simulink model "InertiaWheelSystemSF"
settings: Solver=ode45  StartTime=0.0  StopTime=10.0  RelTol=1e-6
values from neighbouring files (symbols this model uses):
  A = [0 1 0; a 0 0; 0 0 0]    [modelinertia.m]    (also in modellinertia.m = [0 1 0 0; a 0 0 0; 0 0 0 1; 0 0 0 0]; modellinertia2.m = [0 1 0 0; a 0 0 0; 0 0 0 1; 0 0 0 0])
  ang = [1 0 0]    [modelinertia.m]
  B = [B_tau B_d]    [modelinertia.m]    (also in modellinertia.m = [0; b1; 0; -b2]; modellinertia2.m)
  C = Call    [modelinertia.m]    (also in modellinertia.m = [1 0 0 0]; modellinertia2.m = [1 0 0 0])
  D = zeros(3,2)    [modelinertia.m]    (also in modellinertia.m = 0; modellinertia2.m = 0)
  ki = 1/20    (= 0.05)    [modelinertia.m]
  Kt = 59.1186    [Cindesign.m]
  L = 0.30    (= 0.3)    [modelinertia.m]    (also in modellinertia.m; modellinertia2.m)
  N = 328.9617    [Cindesign.m]
  Tdt = 4.4053    [Cindesign.m]
  Tit = 72.0271    [Cindesign.m]
  x10 = 0    [SysInit.m]
  x20 = 0    [SysInit.m]
  x30 = 0    [SysInit.m]
libraries: simulink x7, cstblocks x2
settings Model: Creator=elt11jke  LastModifiedBy=frt090_B
settings DataIOCC: LimitDataPoints=on  SaveFormat=Array  SignalLoggingSaveFormat=ModelDataLogs  ReturnWorkspaceOutputs=off
settings OptimizationCC: ExpressionDepthLimit=2147483647  LifeSpan=inf  SimCompilerOptimization=Off
settings DebuggingCC: UnderspecifiedInitializationDetection=Classic  MergeDetectMultiDrivingBlocksExec=none  SolverPrmCheckMsg=warning  MultiTaskDSMMsg=warning  MultiTaskCondExecSysMsg=none  FcnCallInpInsideContextMsg=Enable All  FrameProcessingCompatibilityMsg=warning  StateNameClashWarn=warning  StrictBusMsg=None  SFUnexpectedBacktrackingDiag=warning  SFNoUnconditionalDefaultTransitionDiag=warning
settings HardwareCC: ProdBitPerPointer=32  ProdLargestAtomicFloat=None  ProdIntDivRoundTo=Undefined  ProdEndianess=Unspecified  ProdWordSize=32  ProdHWDeviceType=32-bit Generic
settings ModelReferenceCC: PropagateSignalLabelsOutOfModel=off
settings SFSimCC: SimUseLocalCustomCode=off
settings RTWCC: RTWUseLocalCustomCode=off  IncludeERTFirstTime=on  RTWCompilerOptimization=Off
settings GRTTargetCC: GeneratePreprocessorConditionals=Disable all

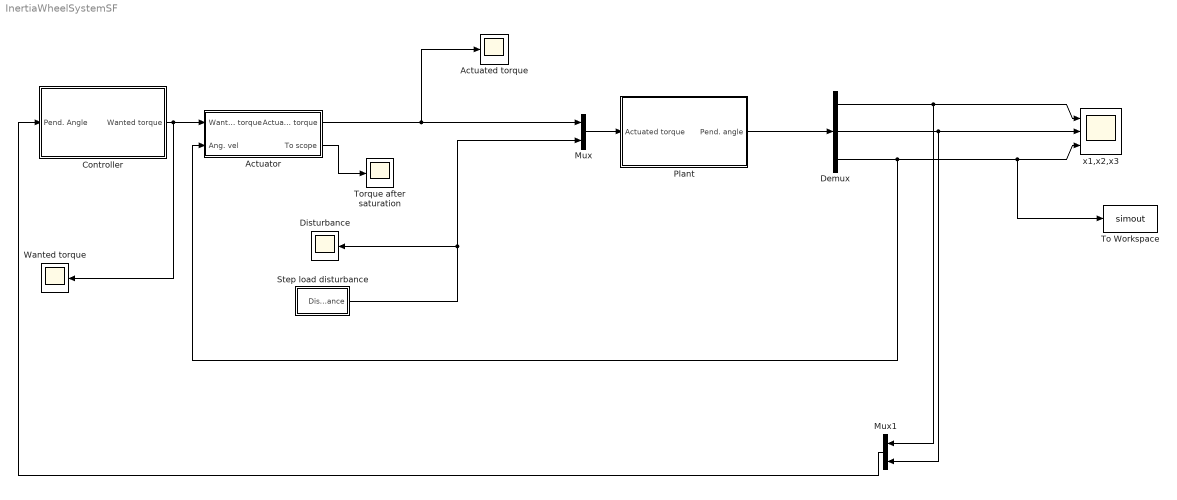
== system InertiaWheelSystemSF ==
  Actuated torque : Scope
      settings: ShowLegends=on  TimeRange=10  YMin=0  YMax=0.00325
  Actuator : Subsystem  TreatAsAtomicUnit=on
  Controller : Subsystem  TreatAsAtomicUnit=on
  Demux : Demux  Outputs=3
  Disturbance : Scope
      settings: ShowLegends=on  TimeRange=10  YMin=-0.01  YMax=0.02  SaveName=ScopeData2
  Mux : Mux  Inputs=2
  Mux1 : Mux  Inputs=2
  Plant : Subsystem  TreatAsAtomicUnit=on
  Step load disturbance : Subsystem
  To Workspace : ToWorkspace  VariableName=simout  SampleTime=-1  SaveFormat=Timeseries
  Torque after saturation : Scope
      settings: ShowLegends=on  TimeRange=10  YMin=0.3648  YMax=0.4032  SaveName=ScopeData4
  Wanted torque : Scope
      settings: ShowLegends=on  TimeRange=10  YMin=-1.355e+07  YMax=-1.3275e+07  SaveName=ScopeData3
  x1,x2,x3 : Scope  NumInputPorts=3
      settings: ShowLegends=on  TimeRange=10  YMin=-6e+38~-6e+39~-20  YMax=2e+38~0~20
  wires:
  Demux/1 -> x1,x2,x3/1, Mux1/1
  Demux/2 -> x1,x2,x3/2, Mux1/2
  Demux/3 -> To Workspace/1, x1,x2,x3/3, Actuator/2(Ang. vel)
  Actuator/2(To scope) -> Torque after saturation/1
  Actuator/1(Actuated torque) -> Mux/1, Actuated torque/1
  Step load disturbance/1(Disturbance) -> Mux/2, Disturbance/1
  Controller/1(Wanted torque) -> Actuator/1(Wanted torque), Wanted torque/1
  Mux/1 -> Plant/1(Actuated torque)
  Plant/1(Pend. angle) -> Demux/1
  Mux1/1 -> Controller/1(Pend. Angle)

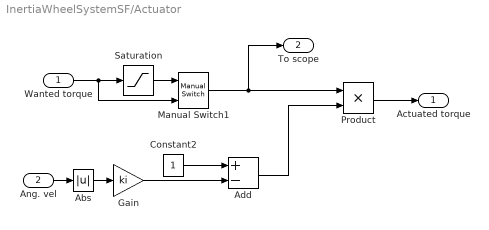
== system InertiaWheelSystemSF/Actuator ==
  Wanted torque : Inport
  Ang. vel : Inport  Port=2
  Abs : Abs
  Add : Sum  Inputs=+-
  Constant2 : Constant
  Gain : Gain  Gain=ki
  Manual Switch1 : simulink/Signal Routing/Manual Switch  sw=1  action=0  varsize=off
  Product : Product  RndMeth=Zero
  Saturation : Saturate  UpperLimit=0.384  LowerLimit=-0.384
  Actuated torque : Outport
  To scope : Outport  Port=2
  wires:
  Wanted torque/1 -> Saturation/1, Manual Switch1/2
  Saturation/1 -> Manual Switch1/1
  Constant2/1 -> Add/1
  Product/1 -> Actuated torque/1
  Add/1 -> Product/2
  Manual Switch1/1 -> Product/1, To scope/1
  Abs/1 -> Gain/1
  Ang. vel/1 -> Abs/1
  Gain/1 -> Add/2

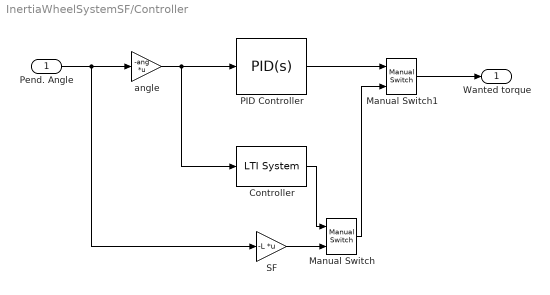
== system InertiaWheelSystemSF/Controller ==
  Pend. Angle : Inport
  Controller : cstblocks/LTI System  sys=Cin  IC=[]
  Manual Switch : simulink/Signal Routing/Manual Switch  sw=0  action=0  varsize=off
  Manual Switch1 : simulink/Signal Routing/Manual Switch  sw=0  action=0  varsize=off
  PID Controller : simulink/Continuous/PID Controller  Controller=PID  TimeDomain=Continuous-time  SampleTime=1  IntegratorMethod=Forward Euler  FilterMethod=Forward Euler  Form=Parallel  P=Kt  I=Tit  D=Tdt  N=N  InitialConditionSource=internal  InitialConditionForIntegrator=0  InitialConditionForFilter=0  ExternalReset=none  LimitOutput=off  UpperSaturationLimit=inf  LowerSaturationLimit=-inf  LinearizeAsGain=off  AntiWindupMode=none  Kb=1  TrackingMode=off  Kt=1  PParamMin=[]  PParamMax=[]  IParamMin=[]  IParamMax=[]  DParamMin=[]  DParamMax=[]  NParamMin=[]  NParamMax=[]  KbParamMin=[]  KbParamMax=[]  KtParamMin=[]  KtParamMax=[]  POutMin=[]  POutMax=[]  IOutMin=[]  IOutMax=[]  DOutMin=[]  DOutMax=[]  NOutMin=[]  NOutMax=[]  KbOutMin=[]  KbOutMax=[]  KtOutMin=[]  KtOutMax=[]  IntegratorOutMin=[]  IntegratorOutMax=[]  FilterOutMin=[]  FilterOutMax=[]  SumOutMin=[]  SumOutMax=[]  SumI1OutMin=[]  SumI1OutMax=[]  SumI2OutMin=[]  SumI2OutMax=[]  SumI3OutMin=[]  SumI3OutMax=[]  SumDOutMin=[]  SumDOutMax=[]  SaturationOutMin=[]  SaturationOutMax=[]  IntegratorContinuousStateAttributes=''  IntegratorStateMustResolveToSignalObject=off  IntegratorRTWStateStorageClass=Auto  FilterContinuousStateAttributes=''  FilterStateMustResolveToSignalObject=off  FilterRTWStateStorageClass=Auto
  SF : Gain  Gain=-L  Multiplication=Matrix(K*u)
  angle : Gain  Gain=-ang  Multiplication=Matrix(K*u)
  Wanted torque : Outport
  wires:
  PID Controller/1 -> Manual Switch1/1
  Manual Switch1/1 -> Wanted torque/1
  Controller/1 -> Manual Switch/1
  Manual Switch/1 -> Manual Switch1/2
  Pend. Angle/1 -> angle/1, SF/1
  angle/1 -> PID Controller/1, Controller/1
  SF/1 -> Manual Switch/2

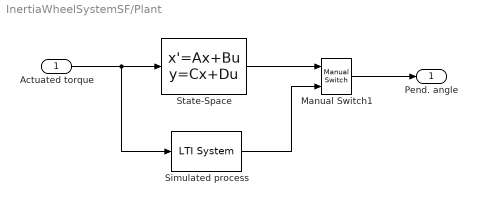
== system InertiaWheelSystemSF/Plant ==
  Actuated torque : Inport
  Manual Switch1 : simulink/Signal Routing/Manual Switch  sw=1  action=0  varsize=off
  Simulated process : cstblocks/LTI System  sys=PinSF  IC=[]
  State-Space : StateSpace  A=A  B=B  C=C  D=D  X0=[x10 x20 x30]
  Pend. angle : Outport
  wires:
  Manual Switch1/1 -> Pend. angle/1
  Actuated torque/1 -> State-Space/1, Simulated process/1
  State-Space/1 -> Manual Switch1/1
  Simulated process/1 -> Manual Switch1/2

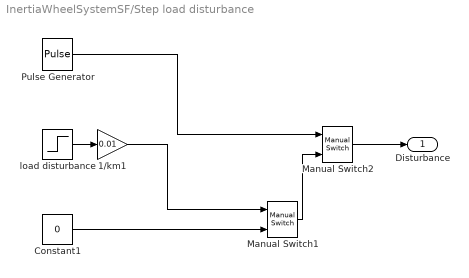
== system InertiaWheelSystemSF/Step load disturbance ==
  1/km1 : Gain  Gain=0.01  SaturateOnIntegerOverflow=on  OutDataTypeStr=Inherit: Same as input  ParamDataTypeStr=Inherit: Same as input
  Constant1 : Constant  Value=0
  Manual Switch1 : simulink/Signal Routing/Manual Switch  sw=0  action=0  varsize=off
  Manual Switch2 : simulink/Signal Routing/Manual Switch  sw=1  action=0  varsize=off
  Pulse Generator : DiscretePulseGenerator  PulseType=Time based  Amplitude=2  Period=3  PulseWidth=10
  load disturbance : Step  Time=5  After=-0.15  SampleTime=0
  Disturbance : Outport
  wires:
  load disturbance/1 -> 1/km1/1
  Constant1/1 -> Manual Switch1/2
  1/km1/1 -> Manual Switch1/1
  Pulse Generator/1 -> Manual Switch2/1
  Manual Switch1/1 -> Manual Switch2/2
  Manual Switch2/1 -> Disturbance/1
